simulink model "Sim_Der3"  (R2021a)
settings: Solver=FixedStepAuto  StartTime=0.0  StopTime=5  FixedStep=Ts  RelTol=1e-3
undefined symbols (not defined in the file): Noise, signal, Ts, TWindow
libraries: simulink x1
settings Model: Creator=perruquetti  LastModifiedBy=perruquetti

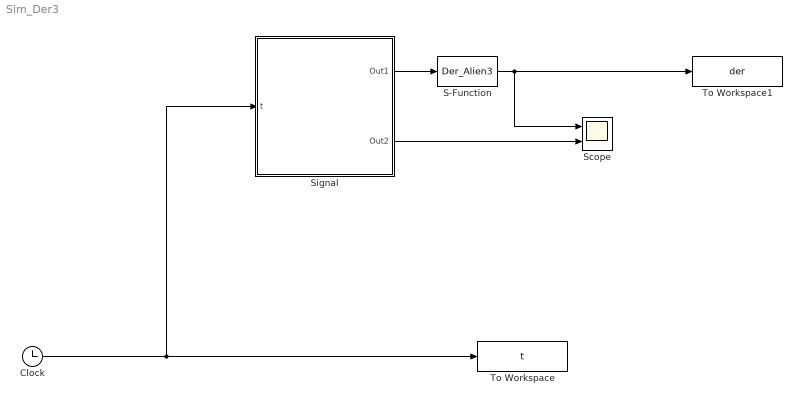
== system Sim_Der3 ==
  Clock : Clock
  S-Function : S-Function  FunctionName=Der_Alien3  Parameters=Ts,TWindow  SFunctionDeploymentMode=off  EnableBusSupport=off
  Scope : Scope  NumInputPorts=2
  Signal : Subsystem
  To Workspace : ToWorkspace  VariableName=t  SampleTime=-1
  To Workspace1 : ToWorkspace  VariableName=der  SampleTime=-1
  wires:
  Clock/1 -> Signal/1(t), To Workspace/1
  S-Function/1 -> Scope/1, To Workspace1/1
  Signal/1(Out1) -> S-Function/1
  Signal/2(Out2) -> Scope/2

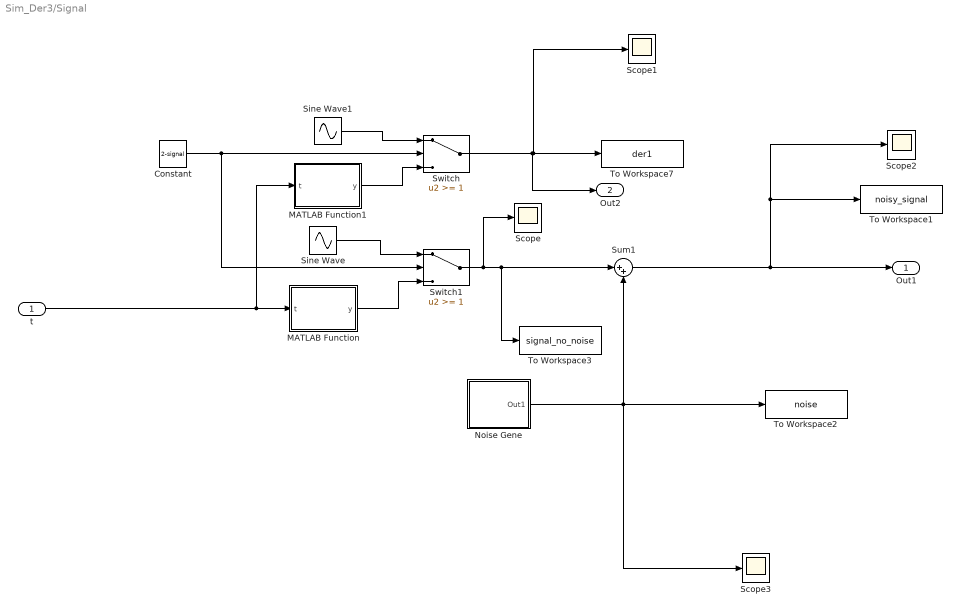
== system Sim_Der3/Signal ==
  t : Inport
  Constant : Constant  Value=2-signal
  MATLAB Function : MATLAB Function  TreatAsAtomicUnit=on
  MATLAB Function1 : MATLAB Function  TreatAsAtomicUnit=on
  Noise Gene : Subsystem
  Scope{,1..3} (4 alike) : Scope
  Sine Wave : Sin  Frequency=10  SampleTime=0
  Sine Wave1 : Sin  Amplitude=10  Frequency=10  Phase=90  SampleTime=0
  Sum1 : Sum  Inputs=|++
  Switch : Switch  Threshold=1
  Switch1 : Switch  Threshold=1
  To Workspace1 : ToWorkspace  VariableName=noisy_signal  SampleTime=-1
  To Workspace2 : ToWorkspace  VariableName=noise  SaveFormat=Timeseries  SampleTime=-1
  To Workspace3 : ToWorkspace  VariableName=signal_no_noise  SampleTime=-1
  To Workspace7 : ToWorkspace  VariableName=der1  SampleTime=-1
  Out1 : Outport
  Out2 : Outport  Port=2
  wires:
  Switch/1 -> Out2/1, Scope1/1, To Workspace7/1
  MATLAB Function1/1(y) -> Switch/3
  Constant/1 -> Switch1/2, Switch/2
  Sine Wave1/1 -> Switch/1
  Noise Gene/1(Out1) -> Scope3/1, Sum1/2, To Workspace2/1
  t/1 -> MATLAB Function1/1(t), MATLAB Function/1(t)
  Sine Wave/1 -> Switch1/1
  MATLAB Function/1(y) -> Switch1/3
  Switch1/1 -> Scope/1, To Workspace3/1, Sum1/1
  Sum1/1 -> Out1/1, Scope2/1, To Workspace1/1

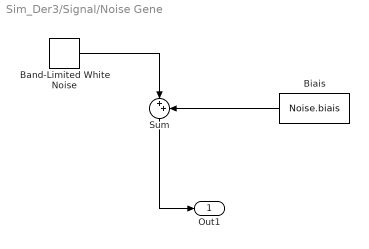
== system Sim_Der3/Signal/Noise Gene ==
  Band-Limited White Noise : simulink/Sources/Band-Limited White Noise  Cov=Noise.power  Ts=Noise.sampling  seed=Noise.seed
  Biais : Constant  Value=Noise.biais
  Sum : Sum  Inputs=|++
  Out1 : Outport
  wires:
  Sum/1 -> Out1/1
  Biais/1 -> Sum/2
  Band-Limited White Noise/1 -> Sum/1

== matlab function Sim_Der3/Signal/MATLAB Function ==
  data: t input; y output
function y = fcn(t)

y = tanh(t-1)+exp(-t/1.2)*sin(6*t+pi);

== matlab function Sim_Der3/Signal/MATLAB Function1 ==
  data: t input; y output
function y = fcn(t)

y = (cosh(t-1))^(-2)+exp(-t/1.2)*(-1/1.2*sin(6*t+pi)+6*cos(6*t+pi));
